simulink model "powerpll"  (Simulink 6.6)
settings: Solver=ode23t  StartTime=0.0  StopTime=50e-6  RelTol=1e-3
PostLoadFcn:
  | C2 = 17e-12;
  | C1 = 82e-12;
  | R1 = 23e3;
libraries: powerlib x13, simulink_extras x2, commsynccomp2 x1
settings Model: Creator=Edwin Pasterkamp  LastModifiedBy=epasterk
settings DebuggingCC: SignalResolutionControl=TryResolveAllWithWarning

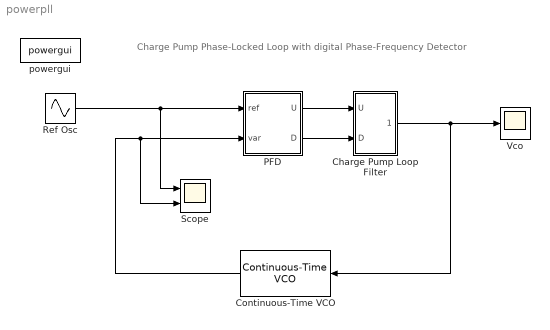
== system powerpll ==
  note: Charge Pump Phase-Locked Loop with digital Phase-Frequency Detector
  Charge Pump Loop Filter : Subsystem
  Continuous-Time VCO : commsynccomp2/Continuous-Time VCO  Orientation=left  SystemSampleTime=-1  Ac=1  Fc=1e6  Kc=10e6/32  Ph=-pi/2
  PFD : Subsystem
  Ref Osc : Sin  Frequency=2*pi*1e6  Phase=pi/2  SampleTime=0
      settings: AttributesFormatString=%<Frequency> (rad/s)
  Scope : Scope  NumInputPorts=2
      settings: TimeRange=5e-005  YMin=-1.5~-1.5  YMax=1.5~1.5  SaveName=ScopeData4  SampleInput=on  SampleTime=1e-8
  Vco : Scope
      settings: TimeRange=0.00012  YMin=-2
  powergui : powerlib/powergui  SystemSampleTime=-1  SimulationMode=Continuous  SampleTime=50e-6  echomessages=off  RestoreLinks=warning  x0status=blocks  Frange=[0:2:500]  Ylog=off  Xlog=on  ShowGrid=off  save=off  variable=ZData  ZoomFFT=on  StartTime=0.0  cycles=1  DisplayStyle=1  fundamental=60  FreqAxis=off  MaxFrequency=1000  frequencyindice=0  frequencyindicesteady=1  RmsSteady=1  display=off  Ts=0  frequency=60  methode=off  HookPort=off  Interpol=off
  wires:
  Ref Osc/1 -> Scope/1, PFD/1(ref)
  Continuous-Time VCO/1 -> Scope/2, PFD/2(var)
  PFD/1(U) -> Charge Pump Loop Filter/1(U)
  PFD/2(D) -> Charge Pump Loop Filter/2(D)
  Charge Pump Loop Filter/1(contrl) -> Continuous-Time VCO/1, Vco/1

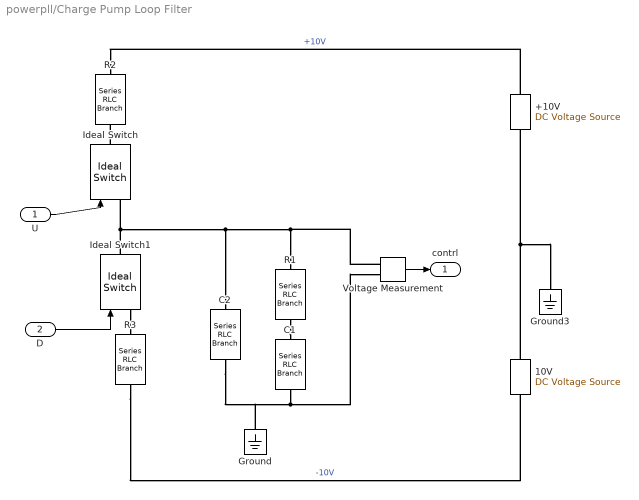
== system powerpll/Charge Pump Loop Filter ==
  U : Inport
  D : Inport  Port=2
  +10V : powerlib/Electrical Sources/DC Voltage Source  Orientation=up  DialogController=POWERSYS.PowerSysDialog  SystemSampleTime=-1  Amplitude=10  Measurements=None
  10V : powerlib/Electrical Sources/DC Voltage Source  Orientation=up  DialogController=POWERSYS.PowerSysDialog  SystemSampleTime=-1  Amplitude=10  Measurements=None
  C1 : powerlib/Elements/Series RLC Branch  Orientation=down  DialogController=POWERSYS.PowerSysDialog  PhysicalDomain=powersysdomain  SubClassName=unknown  LeftPortType=p1  RightPortType=p1  LConnTagsString=__new0  RConnTagsString=__new0  BranchType=C  Resistance=1  Inductance=1e-3  SetiL0=off  InitialCurrent=0  Capacitance=C1  Setx0=off  InitialVoltage=0  Measurements=None
  C2 : powerlib/Elements/Series RLC Branch  Orientation=down  DialogController=POWERSYS.PowerSysDialog  PhysicalDomain=powersysdomain  SubClassName=unknown  LeftPortType=p1  RightPortType=p1  LConnTagsString=__new0  RConnTagsString=__new0  BranchType=C  Resistance=1  Inductance=1e-3  SetiL0=off  InitialCurrent=0  Capacitance=C2  Setx0=off  InitialVoltage=0  Measurements=None
  Ground : powerlib/Elements/Ground  Orientation=down  DialogController=POWERSYS.PowerSysDialog  PhysicalDomain=powersysdomain  SubClassName=unknown  LeftPortType=p1  RightPortType=p1  LConnTagsString=a
  Ground3 : powerlib/Elements/Ground  Orientation=down  DialogController=POWERSYS.PowerSysDialog  PhysicalDomain=powersysdomain  SubClassName=unknown  LeftPortType=p1  RightPortType=p1  LConnTagsString=a
  Ideal Switch : powerlib/Power Electronics/Ideal Switch  Orientation=up  DialogController=POWERSYS.PowerSysDialog  SystemSampleTime=-1  Ron=0.001  Lon=0  IC=0  Rs=1e8  Cs=inf  Measurements=off
  Ideal Switch1 : powerlib/Power Electronics/Ideal Switch  Orientation=up  DialogController=POWERSYS.PowerSysDialog  SystemSampleTime=-1  Ron=0.001  Lon=0  IC=0  Rs=1e8  Cs=inf  Measurements=off
  R1 : powerlib/Elements/Series RLC Branch  Orientation=down  DialogController=POWERSYS.PowerSysDialog  PhysicalDomain=powersysdomain  SubClassName=unknown  LeftPortType=p1  RightPortType=p1  LConnTagsString=__new0  RConnTagsString=__new0  BranchType=R  Resistance=R1  Inductance=1e-3  SetiL0=off  InitialCurrent=0  Capacitance=C1  Setx0=off  InitialVoltage=0  Measurements=None
  R2 : powerlib/Elements/Series RLC Branch  Orientation=down  DialogController=POWERSYS.PowerSysDialog  PhysicalDomain=powersysdomain  SubClassName=unknown  LeftPortType=p1  RightPortType=p1  LConnTagsString=__new0  RConnTagsString=__new0  BranchType=R  Resistance=40e3  Inductance=1e-3  SetiL0=off  InitialCurrent=0  Capacitance=C1  Setx0=off  InitialVoltage=0  Measurements=None
  R3 : powerlib/Elements/Series RLC Branch  Orientation=down  DialogController=POWERSYS.PowerSysDialog  PhysicalDomain=powersysdomain  SubClassName=unknown  LeftPortType=p1  RightPortType=p1  LConnTagsString=__new0  RConnTagsString=__new0  BranchType=R  Resistance=40e3  Inductance=1e-3  SetiL0=off  InitialCurrent=0  Capacitance=C1  Setx0=off  InitialVoltage=0  Measurements=None
  Voltage Measurement : powerlib/Measurements/Voltage Measurement  DialogController=POWERSYS.PowerSysDialog  SystemSampleTime=-1  PhasorSimulation=off  OutputType=Complex  PSBequivalent=0
  contrl : Outport
  wires:
  D/1 -> Ideal Switch1/1
  Voltage Measurement/1 -> contrl/1
  U/1 -> Ideal Switch/1
  connections:
  R1/RConn1 -- C1/LConn1
  C1/RConn1 -- Ground/LConn1 -- C2/RConn1 -- Voltage Measurement/LConn2
  Ideal Switch1/RConn1 -- C2/LConn1 -- R1/LConn1 -- Voltage Measurement/LConn1 -- Ideal Switch/LConn1
  R3/RConn1 -- 10V/LConn1  "-10V"
  Ideal Switch1/LConn1 -- R3/LConn1
  Ideal Switch/RConn1 -- R2/RConn1
  10V/RConn1 -- +10V/LConn1 -- Ground3/LConn1
  +10V/RConn1 -- R2/LConn1  "+10V"

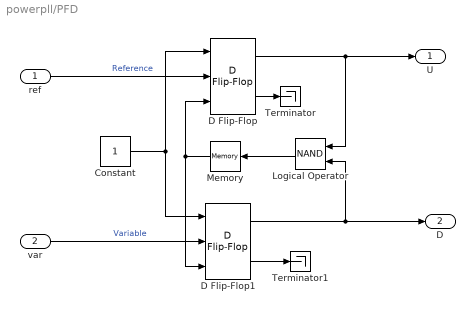
== system powerpll/PFD ==
  ref : Inport
  var : Inport  Port=2
  Constant : Constant  OutDataTypeMode=boolean
  D Flip-Flop : simulink_extras/Flip Flops/D Flip-Flop  SystemSampleTime=-1
  D Flip-Flop1 : simulink_extras/Flip Flops/D Flip-Flop  SystemSampleTime=-1
  Logical Operator : Logic  Orientation=left  Operator=NAND
  Memory : Memory  Orientation=left
  Terminator : Terminator
  Terminator1 : Terminator
  U : Outport
  D : Outport  Port=2
  wires:
  D Flip-Flop/2 -> Terminator/1
  D Flip-Flop1/2 -> Terminator1/1
  Logical Operator/1 -> Memory/1
  ref/1 -> D Flip-Flop/2  "Reference"
  var/1 -> D Flip-Flop1/2  "Variable"
  Constant/1 -> D Flip-Flop/1, D Flip-Flop1/1
  Memory/1 -> D Flip-Flop/3, D Flip-Flop1/3
  D Flip-Flop/1 -> U/1, Logical Operator/1
  D Flip-Flop1/1 -> D/1, Logical Operator/2
